simulink model "TD"  (R2022b)
settings: Solver=VariableStepAuto  StartTime=0.0  StopTime=200000  RelTol=1e-3
undefined symbols (not defined in the file): h
settings Model: Creator=liaoy  LastModifiedBy=liaoy

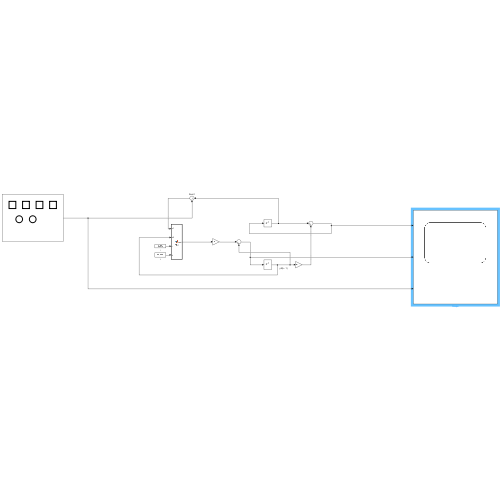
[thumbnail: Simulink's stored preview of the top-level diagram]
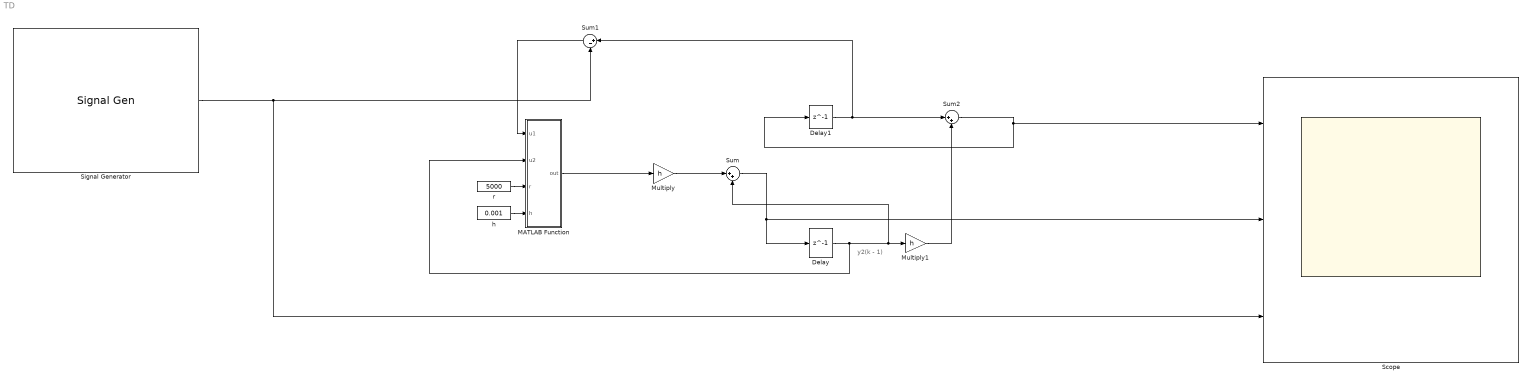
== system TD ==
  note: y2(k - 1)
  Delay : Delay  DelayLength=1  InitialCondition=0  SampleTime=80
  Delay1 : Delay  DelayLength=1  InitialCondition=0  SampleTime=80
  MATLAB Function : MATLAB Function  TreatAsAtomicUnit=on
  Multiply : Gain  Gain=h
  Multiply1 : Gain  Gain=h
  Scope : Scope  NumInputPorts=3
  Signal Generator : SignalGenerator  WaveForm=random  Amplitude=20  Frequency=0.00001
  Sum : Sum  Inputs=|++
  Sum1 : Sum  Inputs=|+-
  Sum2 : Sum  Inputs=|++
  h : Constant  Value=0.001
  r : Constant  Value=5000
  wires:
  r/1 -> MATLAB Function/3(r)
  h/1 -> MATLAB Function/4(h)
  MATLAB Function/1(out) -> Multiply/1
  Multiply/1 -> Sum/1
  Signal Generator/1 -> Scope/3, Sum1/2
  Sum1/1 -> MATLAB Function/1(u1)
  Sum/1 -> Delay/1, Scope/2
  Delay/1 -> MATLAB Function/2(u2), Sum/2, Multiply1/1
  Delay1/1 -> Sum1/1, Sum2/1
  Multiply1/1 -> Sum2/2
  Sum2/1 -> Delay1/1, Scope/1

== matlab function TD/MATLAB Function ==
  data: u1 input; out output; u2 input; r input; h input
function out = hfst(u1,u2,r,h)
d=r*h;
d0=h*d;
y=u1+h*u2;
a0=sqrt(d*d+8*r*abs(y));
a=0;
out1=0;
if abs(y)>d0
    a=u2+(a0-d)/2*sign(y);
end
 
if abs(y)<=d0
    a=u2+y/h;
end
 
if abs(a)>d
    out1=-r*sign(a);
end
 
if abs(a)<=d
    out1=-r*a/d;
end
out=out1;
end
